simulink model "IonSatSimulationA"  (R2020b)
settings: Solver=ode3  StartTime=0.0  StopTime=t_sim  FixedStep=TimeStep  MaxStep=30  MinStep=.1  RelTol=1e-3
model workspace (MAT data in the model file):
  repartition_matrix : Simulink.Parameter (value not decoded)
  wheel_number : Simulink.Parameter (value not decoded)
values from neighbouring files (symbols this model uses):
  LOAS =     [LOAS.mat]
  MODE = 2    [main_ADCS.m]    (also in main_ADCSv1.m)
  nmax = 2    [main_ADCS.m]    (also in main_ADCSv1.m)
  Use_IGRF = 1    [main_ADCS.m]    (also in main_ADCSv1.m)
  Use_IGRF_KF = 1    [main_ADCS.m]    (also in main_ADCSv1.m)
undefined symbols (not defined in the file or in its folder): att, date, deg, DipoleMod, DiscIntNeverNeededParam, km, m, orbit, rad, s, sat
libraries: aerolibutil x29, aerolibconvert2 x13, vrlib x13, simulink x10, sharedtransform x8, dspmathops x6, sharedutil x4, aerolibobsolete x3, simulink_extras x2, aerolibcelestial x2, dspstat3 x1, aerolibatmos2 x1
(part 2 of 3)

== system IonSatSimulationA/Disturbance Torques /Extract Vect ==
  Qr : Inport
  Demux : Demux
  Mux1 : Mux  Inputs=3
  Product : Product
  Reshape : Reshape  OutputDimensionality=Column vector (2-D)
  Sign : Signum
  Qvect : Outport  VectorParamsAs1DForOutWhenUnconnected=off
  wires:
  Demux/2 -> Mux1/1
  Demux/4 -> Mux1/3
  Demux/3 -> Mux1/2
  Demux/1 -> Sign/1
  Qr/1 -> Demux/1
  Mux1/1 -> Product/2
  Product/1 -> Reshape/1
  Sign/1 -> Product/1
  Reshape/1 -> Qvect/1

== system IonSatSimulationA/IGRF Computation block/Obtain B_ECI ==
  In1 : Inport
  Dipole Subsystem : Subsystem  TreatAsAtomicUnit=on
  IGRF Subsystem : Subsystem  TreatAsAtomicUnit=on
  If : If
  Merge : Merge
  Use_IGRF : Constant  Value=Use_IGRF
  Out1 : Outport  VectorParamsAs1DForOutWhenUnconnected=off
  wires:
  If/1 -> IGRF Subsystem/Action
  In1/1 -> Dipole Subsystem/1(In1), IGRF Subsystem/1(In1)
  IGRF Subsystem/1(Out1) -> Merge/1
  Use_IGRF/1 -> If/1
  Merge/1 -> Out1/1
  Dipole Subsystem/1("B_ECI ") -> Merge/2
  If/2 -> Dipole Subsystem/Action

== system IonSatSimulationA/Kalman Filter/Coarse Sun Sensor ==
  Sat-Sun_ECI : Inport
  SunMeasure : TriggerPort  TriggerType=function-call  IsSimulinkFunction=on  FunctionName=SunMeasureCoarse  FunctionVisibility=scoped  VariantControl=(inherit)
  Demux : Demux  Outputs=2
  Quaternion Rotation1 : aerolibutil/Quaternion Rotation
  Terminator : Terminator
  u : ArgIn  DisableCoverage=on  PortDimensions=7  ArgumentName=u
  y : ArgOut  DisableCoverage=on  PortDimensions=3  ArgumentName=y
  wires:
  Quaternion Rotation1/1 -> y/1  "Sat_Sun_body"
  Sat-Sun_ECI/1 -> Quaternion Rotation1/2
  Demux/2 -> Terminator/1
  Demux/1 -> Quaternion Rotation1/1
  u/1 -> Demux/1

== system IonSatSimulationA/Kalman Filter/Cubesense (Sun Sensor) ==
  Sat-Sun_ECI : Inport
  SunMeasure : TriggerPort  TriggerType=function-call  IsSimulinkFunction=on  FunctionName=SunMeasure  FunctionVisibility=scoped  VariantControl=(inherit)
  Demux : Demux  Outputs=2
  Quaternion Rotation1 : aerolibutil/Quaternion Rotation
  Terminator : Terminator
  u : ArgIn  DisableCoverage=on  PortDimensions=7  ArgumentName=u
  y : ArgOut  DisableCoverage=on  PortDimensions=3  ArgumentName=y
  wires:
  Quaternion Rotation1/1 -> y/1  "Sat_Sun_body"
  Sat-Sun_ECI/1 -> Quaternion Rotation1/2
  Demux/2 -> Terminator/1
  Demux/1 -> Quaternion Rotation1/1
  u/1 -> Demux/1

== system IonSatSimulationA/Kalman Filter/Gyrometer ==
  GyroMeasure : TriggerPort  TriggerType=function-call  IsSimulinkFunction=on  FunctionName=GyroMeasure  FunctionVisibility=scoped  VariantControl=(inherit)
  Demux : Demux  Outputs=2
  Terminator : Terminator
  u : ArgIn  DisableCoverage=on  PortDimensions=7  ArgumentName=u
  y : ArgOut  DisableCoverage=on  PortDimensions=3  ArgumentName=y
  wires:
  u/1 -> Demux/1
  Demux/2 -> y/1  "W_ECI"
  Demux/1 -> Terminator/1  "Q"

== system IonSatSimulationA/Kalman Filter/IGRF Computation block orig ==
  <XYZ_ECI> : Inport
  "DCM_i2e " : Inport  Port=2
  "Time_UTC " : Inport  Port=3
  Bus Creator : BusCreator  Inputs=5
  Bus Selector4 : BusSelector  OutputSignals=XYZ_ECI
  Demux : Demux  Outputs=2
  ECI To LLA : MATLAB Function  TreatAsAtomicUnit=on
  Obtain B_ECI : Subsystem
  Product : Product  Multiplication=Matrix(*)
  Reshape : Reshape  OutputDimensionality=Row vector (2-D)
  Terminator : Terminator
  B_ECI : Outport  VectorParamsAs1DForOutWhenUnconnected=off
  wires:
  ECI To LLA/3(long) -> Bus Creator/3
  ECI To LLA/2(lat) -> Bus Creator/2
  ECI To LLA/1(h) -> Bus Creator/1
  Demux/1 -> Bus Creator/4
  Demux/2 -> Terminator/1
  "DCM_i2e "/1 -> Product/2, Bus Creator/5  "DCM_i2e"
  <XYZ_ECI>/1 -> Bus Selector4/1
  Reshape/1 -> Product/1
  Product/1 -> ECI To LLA/1(X_ECEF)
  Bus Selector4/1 -> Reshape/1  "<XYZ_ECI>"
  Bus Creator/1 -> Obtain B_ECI/1(In1)
  Obtain B_ECI/1(Out1) -> B_ECI/1
  "Time_UTC "/1 -> Demux/1

== system IonSatSimulationA/Kalman Filter/IGRF Computation block1 ==
  <XYZ_ECI> : Inport
  "DCM_i2e " : Inport  Port=2
  "Time_UTC " : Inport  Port=3
  Bus Creator : BusCreator  Inputs=5
  Bus Selector4 : BusSelector  OutputSignals=XYZ_ECI
  Demux : Demux  Outputs=2
  ECI To LLA : MATLAB Function  TreatAsAtomicUnit=on
  Obtain B_ECI : Subsystem
  Product : Product  Multiplication=Matrix(*)
  Reshape : Reshape  OutputDimensionality=Row vector (2-D)
  Terminator : Terminator
  B_ECI : Outport  VectorParamsAs1DForOutWhenUnconnected=off
  wires:
  ECI To LLA/3(long) -> Bus Creator/3
  ECI To LLA/2(lat) -> Bus Creator/2
  ECI To LLA/1(h) -> Bus Creator/1
  Demux/1 -> Bus Creator/4
  Demux/2 -> Terminator/1
  "DCM_i2e "/1 -> Product/2, Bus Creator/5  "DCM_i2e"
  <XYZ_ECI>/1 -> Bus Selector4/1
  Reshape/1 -> Product/1
  Product/1 -> ECI To LLA/1(X_ECEF)
  Bus Selector4/1 -> Reshape/1  "<XYZ_ECI>"
  Bus Creator/1 -> Obtain B_ECI/1(In1)
  Obtain B_ECI/1(Out1) -> B_ECI/1
  "Time_UTC "/1 -> Demux/1

== system IonSatSimulationA/Kalman Filter/Magnetometer ==
  B_IGRFemb_ECI : Inport
  MagMeasure : TriggerPort  TriggerType=function-call  IsSimulinkFunction=on  FunctionName=MagMeasure  FunctionVisibility=scoped  VariantControl=(inherit)
  Demux : Demux  Outputs=2
  Quaternion Rotation : aerolibutil/Quaternion Rotation
  Terminator : Terminator
  u : ArgIn  DisableCoverage=on  PortDimensions=7  ArgumentName=u
  y : ArgOut  DisableCoverage=on  PortDimensions=3  ArgumentName=y
  wires:
  u/1 -> Demux/1
  B_IGRFemb_ECI/1 -> Quaternion Rotation/2
  Demux/2 -> Terminator/1
  Quaternion Rotation/1 -> y/1  "B_IGRF_body"
  Demux/1 -> Quaternion Rotation/1

== system IonSatSimulationA/Kalman Filter/Sat Attitude ==
  OmegaWheels_C : Inport
  dOmegaWheels/dt : Inport  Port=2
  Magnetotorquers_C : Inport  Port=3
  B_IGRFemb_ECI : Inport  Port=4
  f : TriggerPort  TriggerType=function-call  IsSimulinkFunction=on  FunctionName=SatAttitudeFull  FunctionVisibility=scoped  VariantControl=(inherit)
  6DOF in ECI frame : Subsystem
  Demux : Demux  Outputs=2
  Magnetorquer physics : Subsystem
  Mux : Mux  Inputs=2
  Quaternion Rotation : aerolibutil/Quaternion Rotation
  u : ArgIn  DisableCoverage=on  PortDimensions=7  ArgumentName=u
  y : ArgOut  DisableCoverage=on  PortDimensions=7  ArgumentName=y
  wires:
  6DOF in ECI frame/2(W_body) -> Mux/2  "W_body"
  Magnetorquer physics/1(Couple (vect)) -> 6DOF in ECI frame/5(Torque_Body)  "Mag_torque"
  OmegaWheels_C/1 -> 6DOF in ECI frame/3(OmegaWheels)
  Demux/2 -> 6DOF in ECI frame/2("Omega_Body ")
  Magnetotorquers_C/1 -> Magnetorquer physics/1(Mag vector command)  "Mag_command"
  Demux/1 -> Quaternion Rotation/1, 6DOF in ECI frame/1(<Q_ECI>)
  B_IGRFemb_ECI/1 -> Quaternion Rotation/2
  Quaternion Rotation/1 -> Magnetorquer physics/2(B_IGRF_body (vecteur))  "B_IGRF_body"
  6DOF in ECI frame/1(Q_ECI) -> Mux/1  "Q_ECI"
  Mux/1 -> y/1
  u/1 -> Demux/1
  dOmegaWheels/dt/1 -> 6DOF in ECI frame/4(dOmegaWheels/dt)

== system IonSatSimulationA/Kalman Filter/Sat Attitude1 ==
  f : TriggerPort  TriggerType=function-call  IsSimulinkFunction=on  FunctionName=SatAttitude  FunctionVisibility=scoped  VariantControl=(inherit)
  Compute Q_ECI : Subsystem
  Demux : Demux  Outputs=2
  Mux : Mux  Inputs=2
  u : ArgIn  DisableCoverage=on  PortDimensions=7  ArgumentName=u
  y : ArgOut  DisableCoverage=on  PortDimensions=7  ArgumentName=y
  wires:
  Mux/1 -> y/1
  u/1 -> Demux/1
  Demux/1 -> Compute Q_ECI/1(<Q_ECI>)
  Demux/2 -> Mux/2, Compute Q_ECI/2(Omega_body)
  Compute Q_ECI/1(Q_ECI) -> Mux/1

== system IonSatSimulationA/Mission/Compute orbit quaternion ==
  <XYZ_ECI> : Inport
  <VxVyVz_ECI> : Inport  Port=2
  3x3 Cross Product : sharedutil/3x3 Cross Product  aMode=aMode
      settings: SourceProductBaseCode=AE,PW,MT,UV,VE,VP
  Direction Cosine Matrix to Quaternions : sharedtransform/Direction Cosine Matrix  to Quaternions  aMode=0  action=None  tolerance=eps(2)
      settings: SourceProductBaseCode=AE,PW,MT,UV,VE,VP
  Gain : Gain
  Gain1 : Gain  Gain=-1
  Normalization : dspmathops/Normalization  NormType=2-norm  Bias=1e-10  NormOver=Each column  Dimension=1  roundingMode=Floor  overflowMode=off  accumDataTypeStr=Inherit: Same as product output  accumLastDataTypeStr=Inherit: Same as product output  outputDataTypeStr=Inherit: Same as product output  outputMin=[]  outputMax=[]  outputLastDataTypeStr=Inherit: Same as product output
  Normalization1 : dspmathops/Normalization  NormType=2-norm  Bias=1e-10  NormOver=Each column  Dimension=1  roundingMode=Floor  overflowMode=off  accumDataTypeStr=Inherit: Same as product output  accumLastDataTypeStr=Inherit: Same as product output  outputDataTypeStr=Inherit: Same as product output  outputMin=[]  outputMax=[]  outputLastDataTypeStr=Inherit: Same as product output
  Quaternion Inverse : aerolibutil/Quaternion Inverse
  Reshape : Reshape  OutputDimensionality=Column vector (2-D)
  Reshape1 : Reshape  OutputDimensionality=Column vector (2-D)
  Vector Concatenate : Concatenate  NumInputs=3  Mode=Multidimensional array  ConcatenateDimension=2
  Q_orbit : Outport  VectorParamsAs1DForOutWhenUnconnected=off
  wires:
  Normalization/1 -> Reshape/1
  Normalization1/1 -> Reshape1/1
  <VxVyVz_ECI>/1 -> Normalization1/1
  Reshape1/1 -> 3x3 Cross Product/1, Vector Concatenate/1
  <XYZ_ECI>/1 -> Normalization/1
  Reshape/1 -> Gain/1
  Gain/1 -> 3x3 Cross Product/2, Vector Concatenate/3
  Direction Cosine Matrix to Quaternions/1 -> Quaternion Inverse/1
  3x3 Cross Product/1 -> Gain1/1
  Gain1/1 -> Vector Concatenate/2
  Quaternion Inverse/1 -> Q_orbit/1
  Vector Concatenate/1 -> Direction Cosine Matrix to Quaternions/1

== system IonSatSimulationA/Mission/Switch Case Action Subsystem ==
  In1 : Inport
  In2 : Inport  Port=2
  Action Port : ActionPort  ActionPortLabel=default:
  Out1 : Outport  VectorParamsAs1DForOutWhenUnconnected=off
  Out2 : Outport  Port=2  VectorParamsAs1DForOutWhenUnconnected=off
  wires:
  In1/1 -> Out1/1
  In2/1 -> Out2/1

== system IonSatSimulationA/Mission/Switch Case Action Subsystem1 ==
  In1 : Inport
  In2 : Inport  Port=2
  Action Port : ActionPort  ActionPortLabel=case [ 5 ]:
  Out1 : Outport  VectorParamsAs1DForOutWhenUnconnected=off
  Out2 : Outport  Port=2  VectorParamsAs1DForOutWhenUnconnected=off
  wires:
  In1/1 -> Out1/1
  In2/1 -> Out2/1

== system IonSatSimulationA/Mission/Switch Case Action Subsystem2 ==
  In1 : Inport
  In2 : Inport  Port=2
  Action Port : ActionPort  ActionPortLabel=case [ 4 ]:
  Out1 : Outport  VectorParamsAs1DForOutWhenUnconnected=off
  Out2 : Outport  Port=2  VectorParamsAs1DForOutWhenUnconnected=off
  wires:
  In1/1 -> Out1/1
  In2/1 -> Out2/1

== system IonSatSimulationA/Mission/Switch Case Action Subsystem3 ==
  In1 : Inport
  In2 : Inport  Port=2
  Action Port : ActionPort  ActionPortLabel=case [ 3 ]:
  Out1 : Outport  VectorParamsAs1DForOutWhenUnconnected=off
  Out2 : Outport  Port=2  VectorParamsAs1DForOutWhenUnconnected=off
  wires:
  In1/1 -> Out1/1
  In2/1 -> Out2/1

== system IonSatSimulationA/Mission/Switch Case Action Subsystem4 ==
  In1 : Inport
  In2 : Inport  Port=2
  Action Port : ActionPort  ActionPortLabel=case [ 2 ]:
  Out1 : Outport  VectorParamsAs1DForOutWhenUnconnected=off
  Out2 : Outport  Port=2  VectorParamsAs1DForOutWhenUnconnected=off
  wires:
  In1/1 -> Out1/1
  In2/1 -> Out2/1

== system IonSatSimulationA/Mission/Switch Case Action Subsystem5 ==
  In1 : Inport
  In2 : Inport  Port=2
  Action Port : ActionPort  ActionPortLabel=case [ 1 ]:
  Out1 : Outport  VectorParamsAs1DForOutWhenUnconnected=off
  Out2 : Outport  Port=2  VectorParamsAs1DForOutWhenUnconnected=off
  wires:
  In1/1 -> Out1/1
  In2/1 -> Out2/1

== system IonSatSimulationA/Mission/Switch Case Action Subsystem6 ==
  In1 : Inport
  In2 : Inport  Port=2
  Action Port : ActionPort  ActionPortLabel=case [ 7 ]:
  Out1 : Outport  VectorParamsAs1DForOutWhenUnconnected=off
  Out2 : Outport  Port=2  VectorParamsAs1DForOutWhenUnconnected=off
  wires:
  In1/1 -> Out1/1
  In2/1 -> Out2/1

== system IonSatSimulationA/Mission/Switch Case Action Subsystem7 ==
  In1 : Inport
  Input1 : Inport  Port=2
  Action Port : ActionPort  ActionPortLabel=case [ 6 ]:
  Out1 : Outport  VectorParamsAs1DForOutWhenUnconnected=off
  Out3 : Outport  Port=2  VectorParamsAs1DForOutWhenUnconnected=off
  wires:
  In1/1 -> Out1/1
  Input1/1 -> Out3/1

== system IonSatSimulationA/Mission/q_rotation_y_pi//2 ==
  z_ECI : Inport
  V_ECI : Inport  Port=2
  Cross Product : vrlib/Utilities/Cross Product
  Product : Product
  Reshape1 : Reshape  OutputDimensionality=Column vector (2-D)
  Vector Concatenate1 : Concatenate  Mode=Multidimensional array
  cos pi/4 : Constant  Value=[sqrt(2)]
  sin pi/4 : Constant  Value=sqrt(2)
  Q_retrograde : Outport  VectorParamsAs1DForOutWhenUnconnected=off
  wires:
  cos pi/4/1 -> Vector Concatenate1/1
  Vector Concatenate1/1 -> Q_retrograde/1
  sin pi/4/1 -> Product/2
  z_ECI/1 -> Cross Product/1
  V_ECI/1 -> Cross Product/2
  Cross Product/1 -> Product/1  "y"
  Reshape1/1 -> Vector Concatenate1/2
  Product/1 -> Reshape1/1

== system IonSatSimulationA/Mission/q_rotation_z_pi ==
  z_ECI : Inport
  Product : Product
  Reshape1 : Reshape  OutputDimensionality=Column vector (2-D)
  Vector Concatenate1 : Concatenate  Mode=Multidimensional array
  cos pi/2 : Constant  Value=[0]
  sin pi/2 : Constant
  Q_retrograde : Outport  VectorParamsAs1DForOutWhenUnconnected=off
  wires:
  cos pi/2/1 -> Vector Concatenate1/1
  Vector Concatenate1/1 -> Q_retrograde/1
  sin pi/2/1 -> Product/2
  z_ECI/1 -> Product/1
  Product/1 -> Reshape1/1
  Reshape1/1 -> Vector Concatenate1/2

== system IonSatSimulationA/Mission/q_sun_aero ==
  note: choix :
      | x selon V
      | z tel que z.GS soit maximisé
  GS_ECI : Inport
  <VxVyVz_ECI> : Inport  Port=2
  Cross Product : vrlib/Utilities/Cross Product
  Direction Cosine Matrix to Quaternions : sharedtransform/Direction Cosine Matrix  to Quaternions  aMode=0  action=None  tolerance=eps(2)
      settings: SourceProductBaseCode=AE,PW,MT,UV,VE,VP
  Dot Product : DotProduct  InputSameDT=on  OutDataTypeStr=Inherit: Inherit via internal rule
  Normalization1 : dspmathops/Normalization  NormType=2-norm  Bias=1e-10  NormOver=Each column  Dimension=1  roundingMode=Floor  overflowMode=off  accumDataTypeStr=Inherit: Same as product output  accumLastDataTypeStr=Inherit: Same as product output  outputDataTypeStr=Inherit: Same as product output  outputMin=[]  outputMax=[]  outputLastDataTypeStr=Inherit: Same as product output
  Normalization2 : dspmathops/Normalization  NormType=2-norm  Bias=1e-10  NormOver=Each column  Dimension=1  roundingMode=Floor  overflowMode=off  accumDataTypeStr=Inherit: Same as product output  accumLastDataTypeStr=Inherit: Same as product output  outputDataTypeStr=Inherit: Same as product output  outputMin=[]  outputMax=[]  outputLastDataTypeStr=Inherit: Same as product output
  Plus : Sum  Inputs=-+
  Product : Product
  Quaternion Inverse : aerolibutil/Quaternion Inverse
  Reshape1 : Reshape  OutputDimensionality=Column vector (2-D)
  Reshape2 : Reshape  OutputDimensionality=Column vector (2-D)
  Reshape3 : Reshape  OutputDimensionality=Column vector (2-D)
  Vector Concatenate : Concatenate  NumInputs=3  Mode=Multidimensional array  ConcatenateDimension=2
  Q_sun_aero : Outport  VectorParamsAs1DForOutWhenUnconnected=off
  wires:
  Quaternion Inverse/1 -> Q_sun_aero/1
  Reshape2/1 -> Vector Concatenate/3, Cross Product/1
  Reshape3/1 -> Vector Concatenate/1, Cross Product/2
  Product/1 -> Plus/1
  Dot Product/1 -> Product/2
  Cross Product/1 -> Reshape1/1  "y"
  Normalization2/1 -> Reshape2/1  "z"
  Plus/1 -> Normalization2/1  "GS-(GS.x)x"
  GS_ECI/1 -> Dot Product/2, Plus/2
  Vector Concatenate/1 -> Direction Cosine Matrix to Quaternions/1
  Direction Cosine Matrix to Quaternions/1 -> Quaternion Inverse/1
  Normalization1/1 -> Dot Product/1, Product/1, Reshape3/1  "x"
  <VxVyVz_ECI>/1 -> Normalization1/1
  Reshape1/1 -> Vector Concatenate/2

== system IonSatSimulationA/Mission/q_sun_sun ==
  note: Choix:
      | z selon GS
      | x tel que x.V soit maximisé
  <VxVyVz_ECI> : Inport
  GS_ECI : Inport  Port=2
  Cross Product1 : vrlib/Utilities/Cross Product
  Direction Cosine Matrix to Quaternions1 : sharedtransform/Direction Cosine Matrix  to Quaternions  aMode=0  action=None  tolerance=eps(2)
      settings: SourceProductBaseCode=AE,PW,MT,UV,VE,VP
  Dot Product1 : DotProduct  InputSameDT=on  OutDataTypeStr=Inherit: Inherit via internal rule
  Normalization3 : dspmathops/Normalization  NormType=2-norm  Bias=1e-10  NormOver=Each column  Dimension=1  roundingMode=Floor  overflowMode=off  accumDataTypeStr=Inherit: Same as product output  accumLastDataTypeStr=Inherit: Same as product output  outputDataTypeStr=Inherit: Same as product output  outputMin=[]  outputMax=[]  outputLastDataTypeStr=Inherit: Same as product output
  Normalization4 : dspmathops/Normalization  NormType=2-norm  Bias=1e-10  NormOver=Each column  Dimension=1  roundingMode=Floor  overflowMode=off  accumDataTypeStr=Inherit: Same as product output  accumLastDataTypeStr=Inherit: Same as product output  outputDataTypeStr=Inherit: Same as product output  outputMin=[]  outputMax=[]  outputLastDataTypeStr=Inherit: Same as product output
  Plus1 : Sum  Inputs=-+
  Product1 : Product
  Quaternion Inverse1 : aerolibutil/Quaternion Inverse
  Reshape4 : Reshape  OutputDimensionality=Column vector (2-D)
  Reshape5 : Reshape  OutputDimensionality=Column vector (2-D)
  Reshape6 : Reshape  OutputDimensionality=Column vector (2-D)
  Vector Concatenate1 : Concatenate  NumInputs=3  Mode=Multidimensional array  ConcatenateDimension=2
  Q_sun_sun : Outport  VectorParamsAs1DForOutWhenUnconnected=off
  wires:
  Quaternion Inverse1/1 -> Q_sun_sun/1
  Dot Product1/1 -> Product1/1
  Reshape6/1 -> Cross Product1/1, Vector Concatenate1/3
  Reshape5/1 -> Cross Product1/2, Vector Concatenate1/1
  <VxVyVz_ECI>/1 -> Dot Product1/1, Plus1/1
  GS_ECI/1 -> Normalization3/1
  Vector Concatenate1/1 -> Direction Cosine Matrix to Quaternions1/1
  Product1/1 -> Plus1/2
  Plus1/1 -> Normalization4/1  "V-(V.z)z"
  Cross Product1/1 -> Reshape4/1  "y"
  Normalization4/1 -> Reshape5/1  "x"
  Normalization3/1 -> Dot Product1/2, Product1/2, Reshape6/1  "z"
  Direction Cosine Matrix to Quaternions1/1 -> Quaternion Inverse1/1
  Reshape4/1 -> Vector Concatenate1/2

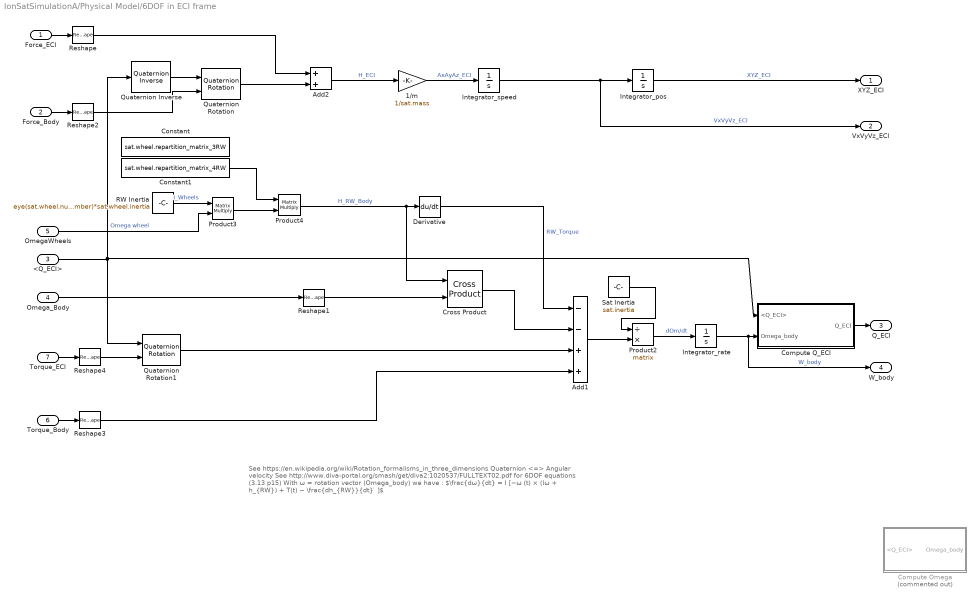
== system IonSatSimulationA/Physical Model/6DOF in ECI frame ==
  note: See https://en.wikipedia.org/wiki/Rotation_formalisms_in_three_dimensions Quaternion <=> Angular velocity
      |
      | See http://www.diva-portal.org/smash/get/diva2:1020537/FULLTEXT02.pdf for 6DOF equations (3.13 p15)
      |
      | With ω = rotation vector (Omega_body) we have :
      |
      | $\frac{dω}{dt} = I [−ω (t) × (Iω + h_{RW}) + T(t) − \frac{dh_{RW}}{dt} ̇ ]$
  Force_ECI : Inport
  Force_Body : Inport  Port=2
  <Q_ECI> : Inport  Port=3
  "Omega_Body " : Inport  Port=4
  OmegaWheels : Inport  Port=5
  Torque_Body : Inport  Port=6
  Torque_ECI : Inport  Port=7  PortDimensions=3
  1/m : Gain  Gain=1/sat.mass
  Add1 : Sum  Inputs=--++
  Add2 : Sum
  Compute Omega : Subsystem  Commented=on
  Compute Q_ECI : Subsystem
  Constant : Constant  Value=sat.wheel.repartition_matrix_3RW
  Constant1 : Constant  Value=sat.wheel.repartition_matrix_4RW
  Cross Product : vrlib/Utilities/Cross Product
  Derivative : Derivative
  Integrator_pos : Integrator
  Integrator_rate : Integrator
  Integrator_speed : Integrator
  Product2 : Product  Inputs=/*  Multiplication=Matrix(*)
  Product3 : Product  Multiplication=Matrix(*)
  Product4 : Product  Multiplication=Matrix(*)
  Quaternion Inverse : aerolibutil/Quaternion Inverse
  Quaternion Rotation : aerolibutil/Quaternion Rotation
  Quaternion Rotation1 : aerolibutil/Quaternion Rotation
  RW Inertia : Constant  Value=eye(sat.wheel.number)*sat.wheel.inertia
  Reshape{,1..4} (5 alike) : Reshape  OutputDimensionality=Column vector (2-D)
  Sat Inertia : Constant  Value=sat.inertia
  XYZ_ECI : Outport  VectorParamsAs1DForOutWhenUnconnected=off
  VxVyVz_ECI : Outport  Port=2  VectorParamsAs1DForOutWhenUnconnected=off
  Q_ECI : Outport  Port=3  VectorParamsAs1DForOutWhenUnconnected=off
  W_body : Outport  Port=4  VectorParamsAs1DForOutWhenUnconnected=off
  wires:
  Product2/1 -> Integrator_rate/1  "dOm/dt"
  Product3/1 -> Product4/2
  Sat Inertia/1 -> Product2/1
  Add1/1 -> Product2/2
  Cross Product/1 -> Add1/2
  "Omega_Body "/1 -> Reshape1/1
  Integrator_rate/1 -> W_body/1, Compute Q_ECI/2(Omega_body)  "W_body"
  RW Inertia/1 -> Product3/1  "I_Wheels"
  Torque_Body/1 -> Reshape3/1
  Derivative/1 -> Add1/1  "RW_Torque"
  OmegaWheels/1 -> Product3/2  "Omega wheel"
  Compute Q_ECI/1(Q_ECI) -> Q_ECI/1
  1/m/1 -> Integrator_speed/1  "AxAyAz_ECI"
  Integrator_pos/1 -> XYZ_ECI/1  "XYZ_ECI"
  Integrator_speed/1 -> VxVyVz_ECI/1, Integrator_pos/1  "VxVyVz_ECI"
  Force_Body/1 -> Reshape2/1
  Quaternion Inverse/1 -> Quaternion Rotation/1
  Add2/1 -> 1/m/1  "H_ECI"
  Quaternion Rotation/1 -> Add2/2
  Force_ECI/1 -> Reshape/1
  Torque_ECI/1 -> Reshape4/1
  <Q_ECI>/1 -> Quaternion Rotation1/1, Quaternion Inverse/1, Compute Q_ECI/1(<Q_ECI>)
  Quaternion Rotation1/1 -> Add1/3
  Constant1/1 -> Product4/1
  Reshape/1 -> Add2/1
  Reshape2/1 -> Quaternion Rotation/2
  Reshape3/1 -> Add1/4
  Reshape4/1 -> Quaternion Rotation1/2
  Product4/1 -> Cross Product/1, Derivative/1  "H_RW_Body"
  Reshape1/1 -> Cross Product/2

== system IonSatSimulationA/Physical Model/Magnetorquer physics ==
  note: On pourrait aussi changer les blocs
      | magnétocoupleurs pour sortir les intensités
  Mag vector command : Inport
  B_IGRF_body (vecteur) : Inport  Port=2
  Add1 : Sum  Inputs=+++
  Cross Product : vrlib/Utilities/Cross Product
  Demux : Demux  Outputs=3
  Magnétocoupleur 1 : Subsystem
  Magnétocoupleur 2 : Subsystem
  Magnétocoupleur 3 : Subsystem
  Couple (vect) : Outport  PortDimensions=3  VectorParamsAs1DForOutWhenUnconnected=off
  Real mag moments vector : Outport  Port=2  VectorParamsAs1DForOutWhenUnconnected=off
  wires:
  Add1/1 -> Real mag moments vector/1, Cross Product/1  "M_real"
  Demux/1 -> Magnétocoupleur 1/1(m_in (scalar))
  Demux/2 -> Magnétocoupleur 2/1(m_in (scalar))
  Demux/3 -> Magnétocoupleur 3/1(m_in (scalar))
  Mag vector command/1 -> Demux/1
  Magnétocoupleur 2/1(m_out (vect)) -> Add1/2
  Magnétocoupleur 1/1(m_out (vect)) -> Add1/1
  Magnétocoupleur 3/1(m_out (vect)) -> Add1/3
  Cross Product/1 -> Couple (vect)/1  "T_body"
  B_IGRF_body (vecteur)/1 -> Cross Product/2

== system IonSatSimulationA/Physical Model/Spherical Harmonic Gravity ==
  note: Slower subsytem because it's too slow
  XYZ_ECI : Inport
  Time_UTC : Inport  Port=2
  ECI to ECEF : MATLABFcn  MATLABFcn=eci2ecef  OutputDimensions=[3;3]  Output1D=off
  Product : Product  Multiplication=Matrix(*)
  Product1 : Product  Inputs=/*  Multiplication=Matrix(*)
  Spherical Harmonic Gravity Model : aerolibgravity2/Spherical Harmonic Gravity Model  units=Metric (MKS)  degree=100  action=Warning  ptype=EGM2008  datafile='aerogmm2b.mat'
      settings: SourceProductBaseCode=AE
  Transpose : Math  Operator=transpose  SignedPower=on  SaturateOnIntegerOverflow=on
  g_ECI (m/s²) : Outport
  DCM_i2e : Outport  Port=2
  wires:
  ECI to ECEF/1 -> DCM_i2e/1, Product1/1, Product/1
  Transpose/1 -> Product1/2
  Product/1 -> Spherical Harmonic Gravity Model/1
  Spherical Harmonic Gravity Model/1 -> Transpose/1
  XYZ_ECI/1 -> Product/2
  Product1/1 -> g_ECI (m/s²)/1
  Time_UTC/1 -> ECI to ECEF/1

== system IonSatSimulationA/Physical Model/Thruster ==
  On/Off (Boolean) : Inport  OutDataTypeStr=boolean
  Constant : Constant  Value=0
  Cross Product : vrlib/Utilities/Cross Product
  If : If  IfExpression=u1
  If Action Subsystem : Subsystem  TreatAsAtomicUnit=on
  If Action Subsystem1 : Subsystem  TreatAsAtomicUnit=on
  Merge : Merge
  Product : Product
  Thruster Force : Constant  Value=sat.thruster.force
  unit vector of thrust : Constant  Value=sat.thruster.dir
  vector G-Thrust point : Constant  Value=sat.thruster.point
  Force (G_sat) : Outport  VectorParamsAs1DForOutWhenUnconnected=off
  Moment (G_sat) : Outport  Port=2  VectorParamsAs1DForOutWhenUnconnected=off
  wires:
  Product/1 -> Force (G_sat)/1, Cross Product/2
  vector G-Thrust point/1 -> Cross Product/1
  unit vector of thrust/1 -> Product/1
  Cross Product/1 -> Moment (G_sat)/1
  Thruster Force/1 -> If Action Subsystem/1(In1)
  On/Off (Boolean)/1 -> If/1
  If/1 -> If Action Subsystem/Action
  If/2 -> If Action Subsystem1/Action
  If Action Subsystem1/1(Out1) -> Merge/2
  If Action Subsystem/1(Out1) -> Merge/1
  Merge/1 -> Product/2
  Constant/1 -> If Action Subsystem1/1(In1)

== system IonSatSimulationA/Sensors/MEMS Gyro ==
  note: Voir ICD sur le CubeControl (pas 100% sur néanmoins)
  U : Inport
  Bus Selector4 : BusSelector  OutputSignals=W_body
  Constant : Constant  Value=[sat.sensors.gyro_bias sat.sensors.gyro_bias sat.sensors.gyro_bias]
  Random Number : RandomNumber  Mean=[0 0 0]  Variance=sat.sensors.mag_sigma*sat.sensors.mag_sigma  Seed=[0 5 355]  SampleTime=1
  Reshape : Reshape  OutputDimensionality=Column vector (2-D)
  Reshape1 : Reshape  OutputDimensionality=Column vector (2-D)
  Sum : Sum  Inputs=|++
  Sum1 : Sum  Inputs=|++
  W_Body_meas : Outport  VectorParamsAs1DForOutWhenUnconnected=off
  wires:
  U/1 -> Bus Selector4/1
  Random Number/1 -> Reshape/1
  Sum/1 -> Sum1/1
  Reshape/1 -> Sum/2  "Noise"
  Bus Selector4/1 -> Sum/1  "<W_body>"
  Sum1/1 -> W_Body_meas/1
  Constant/1 -> Reshape1/1
  Reshape1/1 -> Sum1/2  "Bias"

== system IonSatSimulationA/Sensors/Magnetometer ==
  note: Valeur constructeur : 1-sigma = 50nT
  U : Inport
  B_IGRF_ECI : Inport  Port=2
  Bus Selector : BusSelector  OutputSignals=Q_ECI
  Quaternion Rotation : aerolibutil/Quaternion Rotation
  Random Number : RandomNumber  Mean=[0 0 0]  Variance=sat.sensors.mag_sigma*sat.sensors.mag_sigma  Seed=[0 5 355]  SampleTime=1
  Reshape : Reshape  OutputDimensionality=Column vector (2-D)
  Sum : Sum  Inputs=|++
  B_Body_meas : Outport  VectorParamsAs1DForOutWhenUnconnected=off
  wires:
  B_IGRF_ECI/1 -> Quaternion Rotation/2
  Random Number/1 -> Reshape/1
  Quaternion Rotation/1 -> Sum/1  "B_IGRF_body"
  Sum/1 -> B_Body_meas/1
  Reshape/1 -> Sum/2
  U/1 -> Bus Selector/1
  Bus Selector/1 -> Quaternion Rotation/1  "<Q_ECI>"

== system IonSatSimulationA/Sensors/Sun Sensor (Coarse) ==
  note: Test d'eclipse (true = soleil visible)
  note: Two sensors because the top-camera has a 3-sigma=0.2° wheread the coarse sun sensors have sigma = 10°
  note: Test d'eclipse
  note: Tests if we are not in eclipse
  Sat-Sun_ECI : Inport
  U : Inport  Port=2
  Bus Selector : BusSelector  OutputSignals=Q_ECI,XYZ_ECI
  Eclipse Test 0: in eclipse 1: illumination : MATLABFcn  MATLABFcn=eclipse_check
  Manual Switch : ManualSwitch
  Mux : Mux  Inputs=2
  Quaternion Rotation : aerolibutil/Quaternion Rotation
  Quaternion Rotation1 : aerolibutil/Quaternion Rotation
  Random Number : RandomNumber  Mean=[0 0 0]  Variance=sat.sensors.sun_coarse_sigma*sat.sensors.sun_coarse_sigma  Seed=[0 5 355]  SampleTime=1  VectorParams1D=off
  Rotation Angles to Quaternions : sharedtransform/Rotation Angles to Quaternions  rotationOrder=ZYX  aMode=aMode
      settings: SourceProductBaseCode=AE,PW,MT,UV,VE,VP
  switch here to never have an eclipse : Constant
  Sat-Sun_coarse_body_meas : Outport  VectorParamsAs1DForOutWhenUnconnected=off
  Sensor active (bool) : Outport  Port=2  VectorParamsAs1DForOutWhenUnconnected=off
  wires:
  Rotation Angles to Quaternions/1 -> Quaternion Rotation/1
  Quaternion Rotation/1 -> Sat-Sun_coarse_body_meas/1
  U/1 -> Bus Selector/1
  Bus Selector/1 -> Quaternion Rotation1/1  "<Q_ECI>"
  Quaternion Rotation1/1 -> Quaternion Rotation/2  "Sat_Sun_body"
  Random Number/1 -> Rotation Angles to Quaternions/1
  Bus Selector/2 -> Mux/1  "<XYZ_ECI>"
  Eclipse Test 0: in eclipse 1: illumination/1 -> Manual Switch/1
  Mux/1 -> Eclipse Test 0: in eclipse 1: illumination/1
  Sat-Sun_ECI/1 -> Mux/2, Quaternion Rotation1/2
  Manual Switch/1 -> Sensor active (bool)/1
  switch here to never have an eclipse/1 -> Manual Switch/2

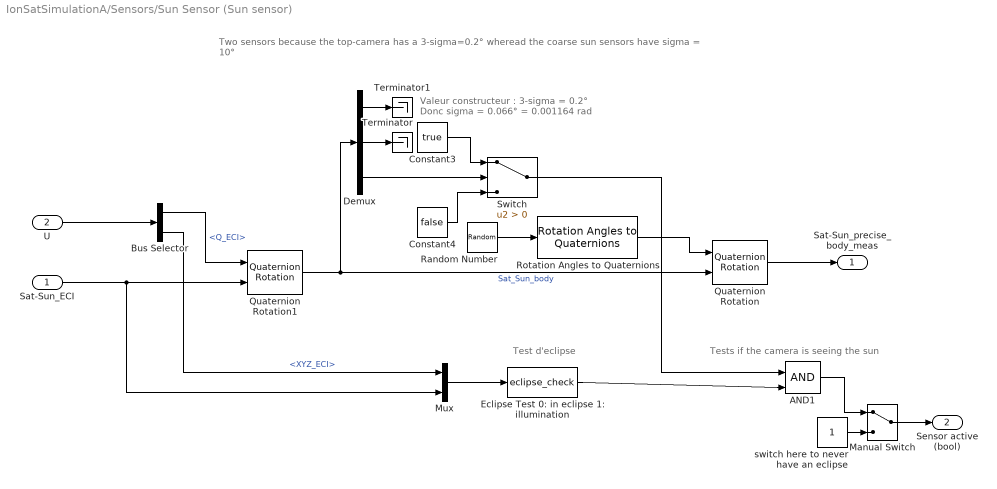
== system IonSatSimulationA/Sensors/Sun Sensor (Sun sensor) ==
  note: Two sensors because the top-camera has a 3-sigma=0.2° wheread the coarse sun sensors have sigma = 10°
  note: Valeur constructeur : 3-sigma = 0.2°
      | Donc sigma = 0.066° = 0.001164 rad
  note: Test d'eclipse
  note: Tests if the camera is seeing the sun
  Sat-Sun_ECI : Inport
  U : Inport  Port=2
  AND1 : Logic  IconShape=distinctive  AllPortsSameDT=off  OutDataTypeStr=boolean
  Bus Selector : BusSelector  OutputSignals=Q_ECI,XYZ_ECI
  Constant3 : Constant  Value=true
  Constant4 : Constant  Value=false
  Demux : Demux  Outputs=3
  Eclipse Test 0: in eclipse 1: illumination : MATLABFcn  MATLABFcn=eclipse_check
  Manual Switch : ManualSwitch
  Mux : Mux  Inputs=2
  Quaternion Rotation : aerolibutil/Quaternion Rotation
  Quaternion Rotation1 : aerolibutil/Quaternion Rotation
  Random Number : RandomNumber  Mean=[0 0 0]  Variance=sat.sensors.sun_sigma*sat.sensors.sun_sigma  Seed=[0 5 355]  SampleTime=1  VectorParams1D=off
  Rotation Angles to Quaternions : sharedtransform/Rotation Angles to Quaternions  rotationOrder=ZYX  aMode=aMode
      settings: SourceProductBaseCode=AE,PW,MT,UV,VE,VP
  Switch : Switch  Criteria=u2 > Threshold
  Terminator : Terminator
  Terminator1 : Terminator
  switch here to never have an eclipse : Constant
  Sat-Sun_precise_body_meas : Outport  VectorParamsAs1DForOutWhenUnconnected=off
  Sensor active (bool) : Outport  Port=2  VectorParamsAs1DForOutWhenUnconnected=off
  wires:
  Rotation Angles to Quaternions/1 -> Quaternion Rotation/1
  Quaternion Rotation/1 -> Sat-Sun_precise_body_meas/1
  U/1 -> Bus Selector/1
  Bus Selector/1 -> Quaternion Rotation1/1  "<Q_ECI>"
  Quaternion Rotation1/1 -> Demux/1, Quaternion Rotation/2  "Sat_Sun_body"
  Demux/3 -> Switch/2
  Constant3/1 -> Switch/1
  Demux/2 -> Terminator/1
  Demux/1 -> Terminator1/1
  Random Number/1 -> Rotation Angles to Quaternions/1
  Constant4/1 -> Switch/3
  Mux/1 -> Eclipse Test 0: in eclipse 1: illumination/1
  AND1/1 -> Manual Switch/1
  Bus Selector/2 -> Mux/1  "<XYZ_ECI>"
  Eclipse Test 0: in eclipse 1: illumination/1 -> AND1/2
  Switch/1 -> AND1/1
  Sat-Sun_ECI/1 -> Mux/2, Quaternion Rotation1/2
  switch here to never have an eclipse/1 -> Manual Switch/2
  Manual Switch/1 -> Sensor active (bool)/1

== system IonSatSimulationA/Attitude Controller/B-dot choice1/Switch Case Action Subsystem3 ==
  In1 : Inport
  Action Port : ActionPort  ActionPortLabel=if(u1 > 0)
  Out1 : Outport  VectorParamsAs1DForOutWhenUnconnected=off
  wires:
  In1/1 -> Out1/1

== system IonSatSimulationA/Attitude Controller/B-dot choice1/Switch Case Action Subsystem4 ==
  In1 : Inport
  Action Port : ActionPort  ActionPortLabel=else
  Out1 : Outport  VectorParamsAs1DForOutWhenUnconnected=off
  wires:
  In1/1 -> Out1/1

== system IonSatSimulationA/Attitude Controller/B-dot choice2/Switch Case Action Subsystem3 ==
  In1 : Inport
  Action Port : ActionPort  ActionPortLabel=if(u1 > 0)
  Out1 : Outport  VectorParamsAs1DForOutWhenUnconnected=off
  wires:
  In1/1 -> Out1/1

== system IonSatSimulationA/Attitude Controller/B-dot choice2/Switch Case Action Subsystem4 ==
  In1 : Inport
  Action Port : ActionPort  ActionPortLabel=else
  Out1 : Outport  VectorParamsAs1DForOutWhenUnconnected=off
  wires:
  In1/1 -> Out1/1

== system IonSatSimulationA/Attitude Controller/PID (nominal command)/Command Magnetic moments computation ==
  note: Moment magnétique de commande M :
      |
      | $M_c = \frac{1}{B²}\vec{B} \wedge\vec{T_P}$
      |
      | Avec Tp couple projeté dans le plan orthogonal à B
      | $T_P=\vec{T}-\frac{1}{B²}(\vec{T}\cdot\vec{B})\vec{B}$
  Command (vect) : Inport  OutDataTypeStr=double
  B_IGRF_body (vect) : Inport  Port=2  OutDataTypeStr=double
  h1 (vect) : Inport  Port=3
  h2 (vect) : Inport  Port=4
  h3 (vect) : Inport  Port=5
  Cross Product : vrlib/Utilities/Cross Product
  Dot Product : DotProduct  InputSameDT=on  OutDataTypeStr=Inherit: Inherit via internal rule
  Global magnetic moment computation : Subsystem
  Mux : Mux  Inputs=3
  Product1 : Product  Inputs=*/
  Reshape : Reshape  OutputDimensionality=Column vector (2-D)
  Reshape1 : Reshape  OutputDimensionality=Column vector (2-D)
  Mag vector command : Outport  VectorParamsAs1DForOutWhenUnconnected=off
  wires:
  B_IGRF_body (vect)/1 -> Reshape1/1  "B_Body"
  Command (vect)/1 -> Reshape/1  "T_Body"
  h1 (vect)/1 -> Global magnetic moment computation/2(In2)
  h2 (vect)/1 -> Global magnetic moment computation/3(In3)
  h3 (vect)/1 -> Global magnetic moment computation/4(In4)
  Global magnetic moment computation/2(magnetic moment 2 (scalar)) -> Mux/2  "magnetic moment 2"
  Global magnetic moment computation/3(magnetic moment 3 (scalar)) -> Mux/3  "magnetic moment 3"
  Global magnetic moment computation/1(magnetic moment 1 (scalar)) -> Mux/1  "magnetic moment 1"
  Mux/1 -> Mag vector command/1
  Reshape1/1 -> Cross Product/2, Dot Product/2, Dot Product/1
  Cross Product/1 -> Product1/1
  Product1/1 -> Global magnetic moment computation/1(In1)  "Mc"
  Dot Product/1 -> Product1/2  "B^2"
  Reshape/1 -> Cross Product/1  "Tp"

== system IonSatSimulationA/Attitude Controller/PID (nominal command)/Extract Vect ==
  Qr : Inport
  Demux : Demux
  Mux1 : Mux  Inputs=3
  Product : Product
  Reshape : Reshape  OutputDimensionality=Column vector (2-D)
  Sign : Signum
  Qvect : Outport  VectorParamsAs1DForOutWhenUnconnected=off
  wires:
  Demux/2 -> Mux1/1
  Demux/4 -> Mux1/3
  Demux/3 -> Mux1/2
  Demux/1 -> Sign/1
  Qr/1 -> Demux/1
  Mux1/1 -> Product/2
  Product/1 -> Reshape/1
  Sign/1 -> Product/1
  Reshape/1 -> Qvect/1

== system IonSatSimulationA/Attitude Controller/PID (nominal command)/If Action Subsystem ==
  In1 : Inport
  Action Port : ActionPort  ActionPortLabel=else
  Out1 : Outport  VectorParamsAs1DForOutWhenUnconnected=off
  wires:
  In1/1 -> Out1/1

== system IonSatSimulationA/Attitude Controller/PID (nominal command)/If Action Subsystem1 ==
  In1 : Inport
  Action Port : ActionPort  ActionPortLabel=if(u1 > 0)
  Out1 : Outport  VectorParamsAs1DForOutWhenUnconnected=off
  wires:
  In1/1 -> Out1/1

== system IonSatSimulationA/Attitude Controller/PID (nominal command)/If Action Subsystem2 ==
  In1 : Inport
  Action Port : ActionPort  ActionPortLabel=if(u1 > 0.0068)
  Out1 : Outport  VectorParamsAs1DForOutWhenUnconnected=off
  wires:
  In1/1 -> Out1/1

== system IonSatSimulationA/Attitude Controller/PID (nominal command)/If Action Subsystem3 ==
  In1 : Inport
  Action Port : ActionPort  ActionPortLabel=else
  Out1 : Outport  VectorParamsAs1DForOutWhenUnconnected=off
  wires:
  In1/1 -> Out1/1

== system IonSatSimulationA/Attitude Controller/PID (nominal command)/RW1 ==
  note: Entrées:
      | - Moment de commande (déjà projeté sur l'axe de la roue...)
      | Sorties:
      | - Omega de commande à appliquer
  Mc (scalar) : Inport
  Discrete-Time Integrator : DiscreteIntegrator  IntegratorMethod=Integration: Trapezoidal  SampleTime=-1  ICPrevOutput=DiscIntNeverNeededParam  ICPrevScaledInput=DiscIntNeverNeededParam
  Divide : Product  Inputs=*/
  Saturation_speed : Saturate  UpperLimit=sat.wheel.max_speed  LowerLimit=- sat.wheel.max_speed
  Torque_sat : Saturate  UpperLimit=sat.wheel.max_torque  LowerLimit=- sat.wheel.max_torque
  Wheel Inertia : Constant  Value=sat.wheel.max_sigma/sat.wheel.max_speed
  Omega_C (scalar) : Outport
  wires:
  Wheel Inertia/1 -> Divide/2
  Divide/1 -> Discrete-Time Integrator/1  "dw/dt"
  Discrete-Time Integrator/1 -> Saturation_speed/1
  Torque_sat/1 -> Divide/1  "Torque (scal)"
  Saturation_speed/1 -> Omega_C (scalar)/1
  Mc (scalar)/1 -> Torque_sat/1

== system IonSatSimulationA/Attitude Controller/PID (nominal command)/RW2 ==
  note: Entrées:
      | - Moment de commande (déjà projeté sur l'axe de la roue...)
      | Sorties:
      | - Omega de commande à appliquer
  Mc (scalar) : Inport
  Discrete-Time Integrator : DiscreteIntegrator  IntegratorMethod=Integration: Trapezoidal  SampleTime=-1  ICPrevOutput=DiscIntNeverNeededParam  ICPrevScaledInput=DiscIntNeverNeededParam
  Divide : Product  Inputs=*/
  Saturation_speed : Saturate  UpperLimit=sat.wheel.max_speed  LowerLimit=- sat.wheel.max_speed
  Torque_sat : Saturate  UpperLimit=sat.wheel.max_torque  LowerLimit=- sat.wheel.max_torque
  Wheel Inertia : Constant  Value=sat.wheel.max_sigma/sat.wheel.max_speed
  Omega_C (scalar) : Outport
  wires:
  Wheel Inertia/1 -> Divide/2
  Divide/1 -> Discrete-Time Integrator/1  "dw/dt"
  Discrete-Time Integrator/1 -> Saturation_speed/1
  Torque_sat/1 -> Divide/1  "Torque (scal)"
  Saturation_speed/1 -> Omega_C (scalar)/1
  Mc (scalar)/1 -> Torque_sat/1

== system IonSatSimulationA/Attitude Controller/PID (nominal command)/RW3 ==
  note: Entrées:
      | - Moment de commande (déjà projeté sur l'axe de la roue...)
      | Sorties:
      | - Omega de commande à appliquer
  Mc (scalar) : Inport
  Discrete-Time Integrator : DiscreteIntegrator  IntegratorMethod=Integration: Trapezoidal  SampleTime=-1  ICPrevOutput=DiscIntNeverNeededParam  ICPrevScaledInput=DiscIntNeverNeededParam
  Divide : Product  Inputs=*/
  Saturation_speed : Saturate  UpperLimit=sat.wheel.max_speed  LowerLimit=- sat.wheel.max_speed
  Torque_sat : Saturate  UpperLimit=sat.wheel.max_torque  LowerLimit=- sat.wheel.max_torque
  Wheel Inertia : Constant  Value=sat.wheel.max_sigma/sat.wheel.max_speed
  Omega_C (scalar) : Outport
  wires:
  Wheel Inertia/1 -> Divide/2
  Divide/1 -> Discrete-Time Integrator/1  "dw/dt"
  Discrete-Time Integrator/1 -> Saturation_speed/1
  Torque_sat/1 -> Divide/1  "Torque (scal)"
  Saturation_speed/1 -> Omega_C (scalar)/1
  Mc (scalar)/1 -> Torque_sat/1

== system IonSatSimulationA/Attitude Controller/PID (nominal command)/RW4  ==
  note: Entrées:
      | - Moment de commande (déjà projeté sur l'axe de la roue...)
      | Sorties:
      | - Omega de commande à appliquer
  Mc (scalar) : Inport
  Discrete-Time Integrator : DiscreteIntegrator  IntegratorMethod=Integration: Trapezoidal  SampleTime=-1  ICPrevOutput=DiscIntNeverNeededParam  ICPrevScaledInput=DiscIntNeverNeededParam
  Divide : Product  Inputs=*/
  Saturation_speed : Saturate  UpperLimit=sat.wheel.max_speed  LowerLimit=- sat.wheel.max_speed
  Torque_sat : Saturate  UpperLimit=sat.wheel.max_torque  LowerLimit=- sat.wheel.max_torque
  Wheel Inertia : Constant  Value=sat.wheel.max_sigma/sat.wheel.max_speed
  Omega_C (scalar) : Outport
  wires:
  Wheel Inertia/1 -> Divide/2
  Divide/1 -> Discrete-Time Integrator/1  "dw/dt"
  Discrete-Time Integrator/1 -> Saturation_speed/1
  Torque_sat/1 -> Divide/1  "Torque (scal)"
  Saturation_speed/1 -> Omega_C (scalar)/1
  Mc (scalar)/1 -> Torque_sat/1

== system IonSatSimulationA/IGRF Computation block/Obtain B_ECI/Dipole Subsystem ==
  In1 : Inport
  Action Port : ActionPort  ActionPortLabel=else
  Bus Selector1 : BusSelector  OutputSignals=h,lat,long,DCM_i2e
  Dipole Model : Subsystem  AncestorBlock=DipoleModel/Dipole Model
  "B_ECI " : Outport  VectorParamsAs1DForOutWhenUnconnected=off
  wires:
  In1/1 -> Bus Selector1/1
  Bus Selector1/1 -> Dipole Model/1(h)  "<h>"
  Bus Selector1/2 -> Dipole Model/2("lat ")  "<lat>"
  Bus Selector1/3 -> Dipole Model/3(long)  "<long>"
  Bus Selector1/4 -> Dipole Model/4(ECI2ECEF_DCM)  "<DCM_i2e>"
  Dipole Model/1("B_ECI ") -> "B_ECI "/1

== system IonSatSimulationA/IGRF Computation block/Obtain B_ECI/IGRF Subsystem ==
  In1 : Inport
  Action Port : ActionPort  ActionPortLabel=if(u1 > 0)
  Bus Selector : BusSelector  OutputSignals=DCM_i2e,h,lat,long,signal4
  International Geomagnetic Reference Field 12 : aerolibobsolete/International Geomagnetic Reference Field 12  units=Metric (MKS)  time_in=on  month=January  day=1  year=2020  action=None  sv_out=on
      settings: SourceProductBaseCode=AE
  Mux : Mux  Inputs=3
  NED to ECEF : MATLABFcn  MATLABFcn=NED2ecef  OutputDimensions=[3;1]  Output1D=off
  Permute Dimensions : PermuteDimensions
  Product : Product  Multiplication=Matrix(*)
  T to nT : Gain  Gain=1E-9
  Terminator{1..9} (9 alike) : Terminator
  Out1 : Outport  VectorParamsAs1DForOutWhenUnconnected=off
  wires:
  In1/1 -> Bus Selector/1
  Bus Selector/2 -> International Geomagnetic Reference Field 12/1  "<h>"
  T to nT/1 -> Out1/1
  Bus Selector/5 -> International Geomagnetic Reference Field 12/4  "<signal4>"
  Bus Selector/4 -> Mux/3, International Geomagnetic Reference Field 12/3  "<long>"
  Bus Selector/3 -> Mux/2, International Geomagnetic Reference Field 12/2  "<lat>"
  International Geomagnetic Reference Field 12/2 -> Terminator1/1
  International Geomagnetic Reference Field 12/10 -> Terminator9/1
  International Geomagnetic Reference Field 12/4 -> Terminator3/1
  International Geomagnetic Reference Field 12/5 -> Terminator4/1
  International Geomagnetic Reference Field 12/3 -> Terminator2/1
  International Geomagnetic Reference Field 12/1 -> Mux/1
  International Geomagnetic Reference Field 12/6 -> Terminator5/1
  International Geomagnetic Reference Field 12/8 -> Terminator7/1
  International Geomagnetic Reference Field 12/7 -> Terminator6/1
  International Geomagnetic Reference Field 12/9 -> Terminator8/1
  Bus Selector/1 -> Permute Dimensions/1  "<DCM_i2e>"
  Permute Dimensions/1 -> Product/1
  Product/1 -> T to nT/1
  Mux/1 -> NED to ECEF/1
  NED to ECEF/1 -> Product/2

== system IonSatSimulationA/Kalman Filter/IGRF Computation block orig/Obtain B_ECI ==
  In1 : Inport
  Dipole Subsystem : Subsystem  TreatAsAtomicUnit=on
  IGRF Subsystem : Subsystem  TreatAsAtomicUnit=on
  If : If
  Merge : Merge
  Use_IGRF : Constant  Value=Use_IGRF_KF
  Out1 : Outport  VectorParamsAs1DForOutWhenUnconnected=off
  wires:
  If/1 -> IGRF Subsystem/Action
  In1/1 -> Dipole Subsystem/1(In1), IGRF Subsystem/1(In1)
  IGRF Subsystem/1(Out1) -> Merge/1
  Use_IGRF/1 -> If/1
  Merge/1 -> Out1/1
  Dipole Subsystem/1(Out1) -> Merge/2
  If/2 -> Dipole Subsystem/Action

== system IonSatSimulationA/Kalman Filter/IGRF Computation block1/Obtain B_ECI ==
  In1 : Inport
  Dipole Subsystem : Subsystem  TreatAsAtomicUnit=on
  IGRF Subsystem : Subsystem  TreatAsAtomicUnit=on
  If : If
  Merge : Merge
  Use_IGRF : Constant  Value=Use_IGRF
  Out1 : Outport  VectorParamsAs1DForOutWhenUnconnected=off
  wires:
  If/1 -> IGRF Subsystem/Action
  In1/1 -> Dipole Subsystem/1(In1), IGRF Subsystem/1(In1)
  IGRF Subsystem/1(Out1) -> Merge/1
  Use_IGRF/1 -> If/1
  Merge/1 -> Out1/1
  Dipole Subsystem/1(Out1) -> Merge/2
  If/2 -> Dipole Subsystem/Action

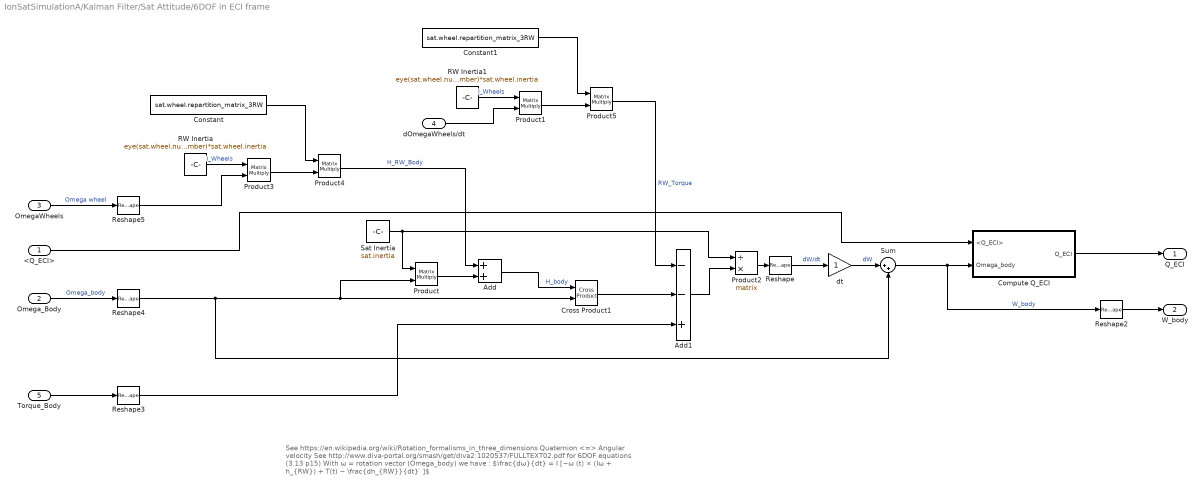
== system IonSatSimulationA/Kalman Filter/Sat Attitude/6DOF in ECI frame ==
  note: See https://en.wikipedia.org/wiki/Rotation_formalisms_in_three_dimensions Quaternion <=> Angular velocity
      |
      | See http://www.diva-portal.org/smash/get/diva2:1020537/FULLTEXT02.pdf for 6DOF equations (3.13 p15)
      |
      | With ω = rotation vector (Omega_body) we have :
      |
      | $\frac{dω}{dt} = I [−ω (t) × (Iω + h_{RW}) + T(t) − \frac{dh_{RW}}{dt} ̇ ]$
  <Q_ECI> : Inport
  "Omega_Body " : Inport  Port=2
  OmegaWheels : Inport  Port=3
  dOmegaWheels/dt : Inport  Port=4
  Torque_Body : Inport  Port=5
  Add : Sum
  Add1 : Sum  Inputs=--+
  Compute Q_ECI : Subsystem
  Constant : Constant  Value=sat.wheel.repartition_matrix_3RW
  Constant1 : Constant  Value=sat.wheel.repartition_matrix_3RW
  Cross Product1 : vrlib/Utilities/Cross Product
  Product{,1,3..5} (5 alike) : Product  Multiplication=Matrix(*)
  Product2 : Product  Inputs=/*  Multiplication=Matrix(*)
  RW Inertia : Constant  Value=eye(sat.wheel.number)*sat.wheel.inertia
  RW Inertia1 : Constant  Value=eye(sat.wheel.number)*sat.wheel.inertia
  Reshape : Reshape
  Reshape2 : Reshape
  Reshape3 : Reshape  OutputDimensionality=Column vector (2-D)
  Reshape4 : Reshape  OutputDimensionality=Column vector (2-D)
  Reshape5 : Reshape  OutputDimensionality=Column vector (2-D)
  Sat Inertia : Constant  Value=sat.inertia
  Sum : Sum  Inputs=|++
  dt : Gain
  Q_ECI : Outport  VectorParamsAs1DForOutWhenUnconnected=off
  W_body : Outport  Port=2  VectorParamsAs1DForOutWhenUnconnected=off
  wires:
  Product2/1 -> Reshape/1
  Product3/1 -> Product4/2
  Sat Inertia/1 -> Product/1, Product2/1
  Add/1 -> Cross Product1/1  "H_body"
  Add1/1 -> Product2/2
  Cross Product1/1 -> Add1/2
  "Omega_Body "/1 -> Reshape4/1  "Omega_body"
  Product/1 -> Add/2
  RW Inertia/1 -> Product3/1  "I_Wheels"
  Torque_Body/1 -> Reshape3/1
  Product5/1 -> Add1/1  "RW_Torque"
  OmegaWheels/1 -> Reshape5/1  "Omega wheel"
  Constant/1 -> Product4/1
  Product4/1 -> Add/1  "H_RW_Body"
  Reshape3/1 -> Add1/3
  Reshape/1 -> dt/1  "dW/dt"
  Sum/1 -> Compute Q_ECI/2(Omega_body), Reshape2/1  "W_body"
  Compute Q_ECI/1(Q_ECI) -> Q_ECI/1
  Reshape2/1 -> W_body/1
  Reshape4/1 -> Sum/2, Cross Product1/2, Product/2
  Reshape5/1 -> Product3/2
  <Q_ECI>/1 -> Compute Q_ECI/1(<Q_ECI>)
  dt/1 -> Sum/1  "dW"
  dOmegaWheels/dt/1 -> Product1/2
  Constant1/1 -> Product5/1
  Product1/1 -> Product5/2
  RW Inertia1/1 -> Product1/1  "I_Wheels"

== system IonSatSimulationA/Kalman Filter/Sat Attitude/Magnetorquer physics ==
  note: On pourrait aussi changer les blocs
      | magnétocoupleurs pour sortir les intensités
  Mag vector command : Inport
  B_IGRF_body (vecteur) : Inport  Port=2
  Add1 : Sum  Inputs=+++
  Cross Product : vrlib/Utilities/Cross Product
  Demux : Demux  Outputs=3
  Magnétocoupleur 1 : Subsystem
  Magnétocoupleur 2 : Subsystem
  Magnétocoupleur 3 : Subsystem
  Couple (vect) : Outport  VectorParamsAs1DForOutWhenUnconnected=off
  wires:
  Add1/1 -> Cross Product/1  "M_real"
  Demux/1 -> Magnétocoupleur 1/1(m_in (scalar))
  Demux/2 -> Magnétocoupleur 2/1(m_in (scalar))
  Demux/3 -> Magnétocoupleur 3/1(m_in (scalar))
  Mag vector command/1 -> Demux/1
  Magnétocoupleur 2/1(m_out (vect)) -> Add1/2
  Magnétocoupleur 1/1(m_out (vect)) -> Add1/1
  Magnétocoupleur 3/1(m_out (vect)) -> Add1/3
  Cross Product/1 -> Couple (vect)/1  "T_body"
  B_IGRF_body (vecteur)/1 -> Cross Product/2

== system IonSatSimulationA/Kalman Filter/Sat Attitude1/Compute Q_ECI ==
  note: https://arxiv.org/pdf/0811.2889.pdf
      | $ω = 2q^*\frac{dq}{dt}$ (13)
      |
      | $\frac{dq}{dt} = \frac{1}{2} q * ω$ (14)
  <Q_ECI> : Inport
  Omega_body : Inport  Port=2
  Gain : Gain  Gain=1/2
  Ground : Ground
  Mux : Mux  Inputs=2
  Quaternion Multiplication : aerolibutil/Quaternion Multiplication
  Quaternion Normalize : sharedutil/Quaternion Normalize  aMode=aMode
      settings: SourceProductBaseCode=AE,PW,MT,UV,VE,VP
  Sum : Sum  Inputs=|++
  dt : Gain
  Q_ECI : Outport  VectorParamsAs1DForOutWhenUnconnected=off
  wires:
  Quaternion Multiplication/1 -> Gain/1
  Omega_body/1 -> Mux/2
  Ground/1 -> Mux/1
  Mux/1 -> Quaternion Multiplication/2
  Quaternion Normalize/1 -> Q_ECI/1  "Q_ECI"
  Sum/1 -> Quaternion Normalize/1
  <Q_ECI>/1 -> Quaternion Multiplication/1, Sum/1
  Gain/1 -> dt/1  "dQ"
  dt/1 -> Sum/2

== system IonSatSimulationA/Physical Model/6DOF in ECI frame/Compute Omega ==
  note: https://arxiv.org/pdf/0811.2889.pdf
      | $ω = 2q^*\frac{dq}{dt}$ (13)
  <Q_ECI> : Inport
  Demux : Demux  Outputs=2
  Derivative : Derivative
  Gain : Gain  Gain=2
  Quaternion Conjugate : aerolibutil/Quaternion Conjugate
      settings: SourceProductBaseCode=AE
  Quaternion Multiplication : aerolibutil/Quaternion Multiplication
  Reshape : Reshape  OutputDimensionality=Column vector (2-D)
  Terminator : Terminator
  Omega_body : Outport  PortDimensions=[3 1]  VectorParamsAs1DForOutWhenUnconnected=off
  wires:
  Quaternion Multiplication/1 -> Demux/1
  <Q_ECI>/1 -> Derivative/1, Quaternion Conjugate/1
  Demux/1 -> Terminator/1
  Demux/2 -> Reshape/1
  Reshape/1 -> Gain/1
  Gain/1 -> Omega_body/1
  Quaternion Conjugate/1 -> Quaternion Multiplication/1
  Derivative/1 -> Quaternion Multiplication/2

== system IonSatSimulationA/Physical Model/6DOF in ECI frame/Compute Q_ECI ==
  note: https://arxiv.org/pdf/0811.2889.pdf
      | $ω = 2q^*\frac{dq}{dt}$ (13)
      |
      | $\frac{dq}{dt} = \frac{1}{2} q * ω$ (14)
  <Q_ECI> : Inport
  Omega_body : Inport  Port=2
  Gain : Gain  Gain=1/2
  Ground : Ground
  Integrator_quat : Integrator  InitialCondition=[1 0 0 0]
  Mux : Mux  Inputs=2
  Quaternion Multiplication : aerolibutil/Quaternion Multiplication
  Quaternion Normalize : sharedutil/Quaternion Normalize  aMode=aMode
      settings: SourceProductBaseCode=AE,PW,MT,UV,VE,VP
  Q_ECI : Outport  VectorParamsAs1DForOutWhenUnconnected=off
  wires:
  Quaternion Multiplication/1 -> Gain/1
  Omega_body/1 -> Mux/2
  Ground/1 -> Mux/1
  Mux/1 -> Quaternion Multiplication/2
  <Q_ECI>/1 -> Quaternion Multiplication/1
  Integrator_quat/1 -> Quaternion Normalize/1
  Gain/1 -> Integrator_quat/1
  Quaternion Normalize/1 -> Q_ECI/1  "Q_ECI"
